simulink model "bic"  (R2014b)
settings: Solver=ode45  StartTime=0.0  StopTime=10.0  RelTol=1e-3
values from neighbouring files (symbols this model uses):
  psi_init = 0    [bicycle.m]
  v_0 = 5    [bicycle.m]
  x_init = 0    [bicycle.m]
  y_init = 0    [bicycle.m]
libraries: simulink x1
settings Model: Creator=Administrator  LastModifiedBy=Administrator

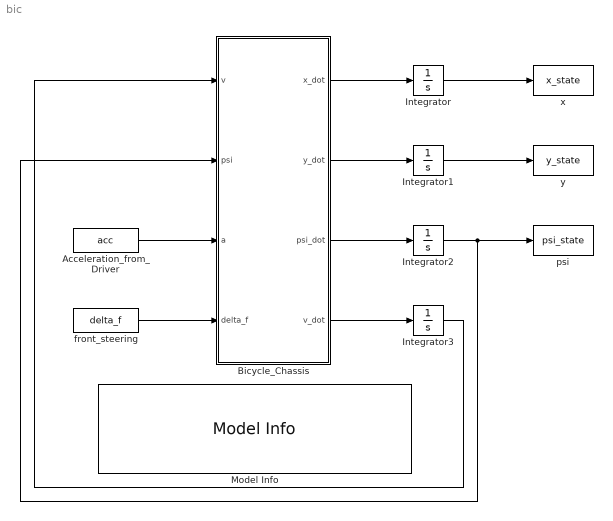
== system bic ==
  " Bicycle_Chassis" : MATLAB Function  TreatAsAtomicUnit=on
  Acceleration_from_Driver : FromWorkspace  VariableName=acc  SampleTime=0
  Integrator : Integrator  InitialCondition=x_init
  Integrator1 : Integrator  InitialCondition=y_init
  Integrator2 : Integrator  InitialCondition=psi_init
  Integrator3 : Integrator  InitialCondition=v_0
  Model Info : simulink/Model-Wide Utilities/Model Info  InitialBlockCM=无  BlockCM=无  Frame=on  DisplayStringWithTags=|  HorizontalTextAlignment=Left  LeftAlignmentValue=0.02  SourceBlockDiagram=bic  TagMaxNumber=20
      | Model Info
      | 
      | [delta_f] is the steering angle on the front wheels.
      | Closewise is Positive.
      | 
      | [acc] is the acceleration requirement.
  front_steering : FromWorkspace  VariableName=delta_f  SampleTime=0
  psi : ToWorkspace  VariableName=psi_state  SampleTime=-1
  x : ToWorkspace  VariableName=x_state  SampleTime=-1
  y : ToWorkspace  VariableName=y_state  SampleTime=-1
  wires:
  " Bicycle_Chassis"/1(x_dot) -> Integrator/1
  " Bicycle_Chassis"/2(y_dot) -> Integrator1/1
  " Bicycle_Chassis"/3(psi_dot) -> Integrator2/1
  " Bicycle_Chassis"/4(v_dot) -> Integrator3/1
  Integrator3/1 -> " Bicycle_Chassis"/1(v)
  Integrator2/1 -> psi/1, " Bicycle_Chassis"/2(psi)
  Integrator/1 -> x/1
  Integrator1/1 -> y/1
  Acceleration_from_Driver/1 -> " Bicycle_Chassis"/3(a)
  front_steering/1 -> " Bicycle_Chassis"/4(delta_f)

== matlab function bic/ Bicycle_Chassis ==
  data: v input; x_dot output; psi input; a input; delta_f input; y_dot output; psi_dot output; v_dot output
function [x_dot,y_dot,psi_dot,v_dot] = bicycle(v, psi,a,delta_f)

lr = 1.6;
lf = 1.4;
wb = lr+lf;
beta = atan(lr/wb*tan(delta_f));

x_dot = v*cos(psi+ beta);
y_dot = v*sin(psi+beta);
psi_dot= v/lr*sin(beta);
v_dot = a;

end

%% ref: http://www.me.berkeley.edu/~frborrel/pdfpub/IV_KinematicMPC_jason.pdf
